simulink library "Radiation_on_Inclined_Surface"  (Simulink 8.2)
settings: Solver=ode45  StartTime=0.0  StopTime=10.0  RelTol=1e-3
libraries: carnot x2
settings Model: Creator=lena.frank  LastModifiedBy=awohlfei

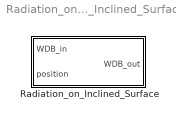
== system Radiation_on_Inclined_Surface ==
  Radiation_on_Inclined_Surface : Subsystem  mask(inclined surface){sky=Perez 1990, reflect=0.2}
      mask prompts: sky "sky model"; reflect "ground reflectance (0..1)"
      mask help: Calculates the radiation on inclined surfaces from sun-position (zenith angle and azimuth). The radiation and incidence angles for the inclined surface are set in the weather vector. All angles are in degrees.
      mask init:
      | reflect = min(1.0, max(0.0, reflect));
      mask Help: web(fullfile(path_carnot('help'),'Radiation_on_Inclined_Surface.html'),'-helpbrowser')
      mask TypeOptions sky: isotropic sky | Hay-Davies | Perez 1990

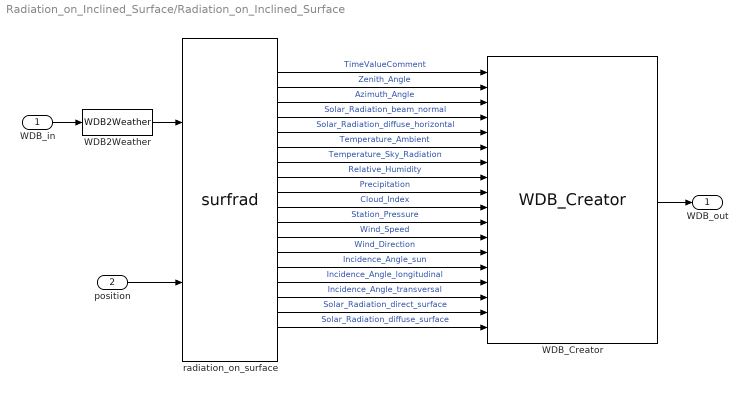
== system Radiation_on_Inclined_Surface/Radiation_on_Inclined_Surface ==
  WDB_in : Inport
  position : Inport  Port=2
  WDB2Weather : carnot/Toolbox/WDB2Weather
  WDB_Creator : carnot/Basic/Weather_and_Sun/WDB_Creator
  radiation_on_surface : S-Function  FunctionName=surfrad  Parameters=sky,reflect  EnableBusSupport=off
  WDB_out : Outport
  wires:
  position/1 -> radiation_on_surface/2
  WDB_in/1 -> WDB2Weather/1
  radiation_on_surface/1 -> WDB_Creator/1  "TimeValueComment"
  radiation_on_surface/2 -> WDB_Creator/2  "Zenith_Angle"
  radiation_on_surface/3 -> WDB_Creator/3  "Azimuth_Angle"
  radiation_on_surface/4 -> WDB_Creator/4  "Solar_Radiation_beam_normal"
  radiation_on_surface/5 -> WDB_Creator/5  "Solar_Radiation_diffuse_horizontal"
  radiation_on_surface/6 -> WDB_Creator/6  "Temperature_Ambient"
  radiation_on_surface/7 -> WDB_Creator/7  "Temperature_Sky_Radiation"
  radiation_on_surface/8 -> WDB_Creator/8  "Relative_Humidity"
  radiation_on_surface/9 -> WDB_Creator/9  "Precipitation"
  radiation_on_surface/10 -> WDB_Creator/10  "Cloud_Index"
  radiation_on_surface/11 -> WDB_Creator/11  "Station_Pressure"
  radiation_on_surface/12 -> WDB_Creator/12  "Wind_Speed"
  radiation_on_surface/13 -> WDB_Creator/13  "Wind_Direction"
  radiation_on_surface/14 -> WDB_Creator/14  "Incidence_Angle_sun"
  radiation_on_surface/15 -> WDB_Creator/15  "Incidence_Angle_longitudinal"
  radiation_on_surface/16 -> WDB_Creator/16  "Incidence_Angle_transversal"
  radiation_on_surface/17 -> WDB_Creator/17  "Solar_Radiation_direct_surface"
  radiation_on_surface/18 -> WDB_Creator/18  "Solar_Radiation_diffuse_surface"
  WDB_Creator/1 -> WDB_out/1
  WDB2Weather/1 -> radiation_on_surface/1
